simulink model "AC_RHP"  (R2022b)
settings: Solver=VariableStepAuto  StartTime=0.0  StopTime=0.5  RelTol=1e-3
undefined symbols (not defined in the file): ac
libraries: acoustical_lib x127, nesl_utility x4
(part 3 of 3)

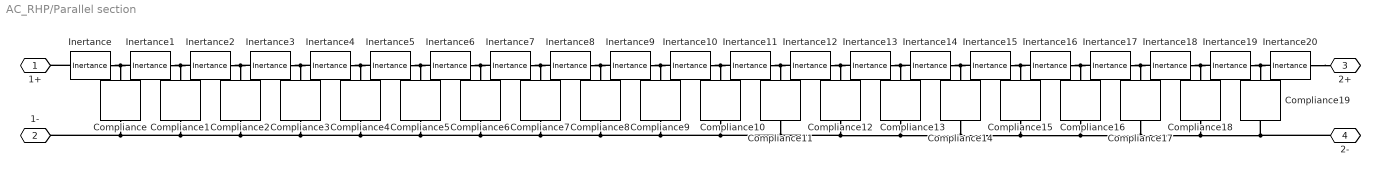
== system AC_RHP/Parallel section ==
  Compliance{,1..19} (20 alike) : acoustical_lib/Acoustical Elements/Compliance  c=ac.ps.C m^3/Pa  r_c=1e-12 Pa/(m^3/s)  g_c=0 m^3/(Pa*s)  u_specify=off  u_priority=None  u=0 m^3/s  u_nominal_specify=off  u_nominal_unit=m^3/s  u_nominal_value=1  p_specify=off  p_priority=None  p=0 Pa  p_nominal_specify=off  p_nominal_unit=Pa  p_nominal_value=1  Pc_specify=off  Pc_priority=High  Pc=0 Pa  Pc_nominal_specify=off  Pc_nominal_unit=Pa  Pc_nominal_value=1
      settings: SourceProductName=Acoustical  InternalSimscapePortConfiguration="{\"Bottom\":[],\"Left\":[{\"id\":\"pp\",\"label\":\"+\",\"type\":\"acoustical.acoustical\"}],\"Right\":[{\"id\":\"nn\",\"label\":\"-\",\"type\":\"acoustical.acoustical\"}],\"Top\":[]}"
  Inertance : acoustical_lib/Acoustical Elements/Inertance  m=ac.ps.L/2 Pa*s^2/m^3  r_m=0 Pa/(m^3/s)  g_m=1e-12 m^3/(Pa*s)  u_specify=off  u_priority=None  u=0 m^3/s  u_nominal_specify=off  u_nominal_unit=m^3/s  u_nominal_value=1  p_specify=off  p_priority=None  p=0 Pa  p_nominal_specify=off  p_nominal_unit=Pa  p_nominal_value=1  U_m_specify=off  U_m_priority=High  U_m=0 m^3/s  U_m_nominal_specify=off  U_m_nominal_unit=m^3/s  U_m_nominal_value=1
      settings: SourceProductName=Acoustical  InternalSimscapePortConfiguration="{\"Bottom\":[],\"Left\":[{\"id\":\"pp\",\"label\":\"+\",\"type\":\"acoustical.acoustical\"}],\"Right\":[{\"id\":\"nn\",\"label\":\"-\",\"type\":\"acoustical.acoustical\"}],\"Top\":[]}"
  Inertance{1..19} (19 alike) : acoustical_lib/Acoustical Elements/Inertance  m=ac.ps.L Pa*s^2/m^3  r_m=0 Pa/(m^3/s)  g_m=1e-12 m^3/(Pa*s)  u_specify=off  u_priority=None  u=0 m^3/s  u_nominal_specify=off  u_nominal_unit=m^3/s  u_nominal_value=1  p_specify=off  p_priority=None  p=0 Pa  p_nominal_specify=off  p_nominal_unit=Pa  p_nominal_value=1  U_m_specify=off  U_m_priority=High  U_m=0 m^3/s  U_m_nominal_specify=off  U_m_nominal_unit=m^3/s  U_m_nominal_value=1
      settings: SourceProductName=Acoustical  InternalSimscapePortConfiguration="{\"Bottom\":[],\"Left\":[{\"id\":\"pp\",\"label\":\"+\",\"type\":\"acoustical.acoustical\"}],\"Right\":[{\"id\":\"nn\",\"label\":\"-\",\"type\":\"acoustical.acoustical\"}],\"Top\":[]}"
  Inertance20 : acoustical_lib/Acoustical Elements/Inertance  m=ac.ps.L/2 Pa*s^2/m^3  r_m=0 Pa/(m^3/s)  g_m=1e-12 m^3/(Pa*s)  u_specify=off  u_priority=None  u=0 m^3/s  u_nominal_specify=off  u_nominal_unit=m^3/s  u_nominal_value=1  p_specify=off  p_priority=None  p=0 Pa  p_nominal_specify=off  p_nominal_unit=Pa  p_nominal_value=1  U_m_specify=off  U_m_priority=High  U_m=0 m^3/s  U_m_nominal_specify=off  U_m_nominal_unit=m^3/s  U_m_nominal_value=1
      settings: SourceProductName=Acoustical  InternalSimscapePortConfiguration="{\"Bottom\":[],\"Left\":[{\"id\":\"pp\",\"label\":\"+\",\"type\":\"acoustical.acoustical\"}],\"Right\":[{\"id\":\"nn\",\"label\":\"-\",\"type\":\"acoustical.acoustical\"}],\"Top\":[]}"
  1+ : PMIOPort  Side=Left
  1- : PMIOPort  Port=2  Side=Left
  2+ : PMIOPort  Port=3  Side=Right
  2- : PMIOPort  Port=4  Side=Right
  connections:
  Inertance19/RConn1 -- Inertance20/LConn1 -- Compliance19/LConn1
  Inertance1/RConn1 -- Inertance2/LConn1 -- Compliance1/LConn1
  Inertance11/RConn1 -- Inertance12/LConn1 -- Compliance11/LConn1
  Inertance/RConn1 -- Inertance1/LConn1 -- Compliance/LConn1
  Inertance7/RConn1 -- Inertance8/LConn1 -- Compliance7/LConn1
  Inertance16/RConn1 -- Inertance17/LConn1 -- Compliance16/LConn1
  Inertance14/RConn1 -- Inertance15/LConn1 -- Compliance14/LConn1
  Inertance18/RConn1 -- Inertance19/LConn1 -- Compliance18/LConn1
  Inertance8/RConn1 -- Inertance9/LConn1 -- Compliance8/LConn1
  Inertance4/RConn1 -- Inertance5/LConn1 -- Compliance4/LConn1
  Inertance3/RConn1 -- Inertance4/LConn1 -- Compliance3/LConn1
  Inertance6/RConn1 -- Inertance7/LConn1 -- Compliance6/LConn1
  Inertance5/RConn1 -- Inertance6/LConn1 -- Compliance5/LConn1
  Inertance2/RConn1 -- Inertance3/LConn1 -- Compliance2/LConn1
  Inertance17/RConn1 -- Inertance18/LConn1 -- Compliance17/LConn1
  Compliance12/LConn1 -- Inertance12/RConn1 -- Inertance13/LConn1
  Inertance13/RConn1 -- Inertance14/LConn1 -- Compliance13/LConn1
  Inertance10/RConn1 -- Inertance11/LConn1 -- Compliance10/LConn1
  Inertance9/RConn1 -- Inertance10/LConn1 -- Compliance9/LConn1
  Inertance15/RConn1 -- Inertance16/LConn1 -- Compliance15/LConn1
  Inertance/LConn1 -- 1+/RConn1
  Inertance20/RConn1 -- 2+/RConn1
  Compliance/RConn1 -- 2-/RConn1 -- Compliance19/RConn1 -- Compliance18/RConn1 -- Compliance17/RConn1 -- Compliance16/RConn1 -- Compliance15/RConn1 -- Compliance14/RConn1 -- Compliance13/RConn1 -- Compliance12/RConn1 -- Compliance11/RConn1 -- Compliance10/RConn1 -- Compliance9/RConn1 -- Compliance8/RConn1 -- Compliance7/RConn1 -- Compliance6/RConn1 -- Compliance5/RConn1 -- Compliance4/RConn1 -- Compliance3/RConn1 -- Compliance2/RConn1 -- Compliance1/RConn1 -- 1-/RConn1
